simulink model "eCS_Old_Algo_And_Tests"  (R2015b)
settings: Solver=VariableStepAuto  StartTime=0.0  StopTime=10.0  RelTol=1e-3
values from neighbouring files (symbols this model uses):
  pulsetype = 2    [Parameter_eCS_Algo.m]    (also in run_simulation.m = j; run_simulation_ActiveX.m = j)
  rotation = 0    [Parameter_eCS_Algo.m]
  SubPulseType = 1    [Parameter_eCS_Algo.m]
undefined symbols (not defined in the file or in its folder): ddv, DiscIntNeverNeededParam, ECE_45_ax, ECE_45_ay, ECE_45_time, gmw_roada_x__m_s__, gmw_roada_y__m_s__, gmw_roadtime_2kHz, Heiko_AY, Heiko_AY_time, Meldorf_HindenburgstraAcceleration_x__m_s_2_, Meldorf_HindenburgstraAcceleration_y__m_s_2_, Meldorf_HindenburgstraTime__s_, pulse_FF27, pulse_MPDB, pulse_ODB40, pulse_ODB64, pulse_USNCAP, pulsetime_FF27, pulsetime_MPDB, pulsetime_ODB40, pulsetime_ODB64, pulsetime_USNCAP, VW_416_2kHza_x_2kHz, VW_416_2kHza_y_2kHz, VW_416_2kHztime_2kHz
libraries: tllib x9, simulink x9
(part 8 of 8)

== system eCS_Old_Algo_And_Tests/eCS_Algo_in_g1/Crash Acceleration/Acceleration Clipping/If Action Subsystem ==
  u8Sample : Inport
  u8OldTrigger : Inport  Port=2
  u8OldTrimer : Inport  Port=3
  Action Port : ActionPort
  "Clear Trigger " : Subsystem  TreatAsAtomicUnit=on
  Decrease Timer : Subsystem  TreatAsAtomicUnit=on
  If1 : If  IfExpression=u1
  Logical Operator : Logic  AllPortsSameDT=off  OutDataTypeStr=boolean  mask(TL_LogicalOperator){data={'date',737938.66931099538}}
      settings: DeleteFcn=if exist('delete_tlblock','file')==2,delete_tlblock(gcbh);end  NameChangeFcn=if exist('rename_tlblock','file')==2,rename_tlblock(gcbh);end  OpenFcn=if exist('tl_open_blockdlg','file')==2,tl_open_blockdlg(gcbh);else,open_system(gcbh,'parameter');end
      mask Help: eval(['if exist(''tl_online_help'',''file'') == 2, tl_online_help(''Topic'',''TL_LogicalOperator''),else, web([''jar:file:///'',matlabroot,''/help/toolbox/simulink/help.jar!/slref/' lower(get_param(gcbh,'Blocktype')) '.html''], ''-helpbrowser''),end'])
      mask Display: plot([-0.1, 1.05, NaN, -0.1, 1.05],[.01, .01, NaN, .99, .99]);
  Logical Operator1 : Logic  AllPortsSameDT=off  OutDataTypeStr=boolean  mask(TL_LogicalOperator){data={'date',737938.66931099538}}
      settings: DeleteFcn=if exist('delete_tlblock','file')==2,delete_tlblock(gcbh);end  NameChangeFcn=if exist('rename_tlblock','file')==2,rename_tlblock(gcbh);end  OpenFcn=if exist('tl_open_blockdlg','file')==2,tl_open_blockdlg(gcbh);else,open_system(gcbh,'parameter');end
      mask Help: eval(['if exist(''tl_online_help'',''file'') == 2, tl_online_help(''Topic'',''TL_LogicalOperator''),else, web([''jar:file:///'',matlabroot,''/help/toolbox/simulink/help.jar!/slref/' lower(get_param(gcbh,'Blocktype')) '.html''], ''-helpbrowser''),end'])
      mask Display: plot([-0.1, 1.05, NaN, -0.1, 1.05],[.01, .01, NaN, .99, .99]);
  MaxSample2 : Constant  Value=ddv('eCS_CFG/CRASH_SAMPLES_NB')  mask(TL_Constant){data={'output',{'variable','eCS_CFG/CRASH_SAMPLES_NB'},'date',737951.42481170141}}
      settings: CopyFcn=if exist('tl_reset_reviewflag') == 2, tl_reset_reviewflag(gcbh); end  DeleteFcn=if exist('delete_tlblock','file')==2,delete_tlblock(gcbh);end  NameChangeFcn=if exist('rename_tlblock','file')==2,rename_tlblock(gcbh);end  OpenFcn=if exist('tl_open_blockdlg','file')==2,tl_open_blockdlg(gcbh);else,open_system(gcbh,'parameter');end
      mask Help: eval(['if exist(''tl_online_help'',''file'') == 2, tl_online_help(''Topic'',''TL_Constant''),else, web([''jar:file:///'',matlabroot,''/help/toolbox/simulink/help.jar!/slref/' lower(get_param(gcbh,'Blocktype')) '.html''], ''-helpbrowser''),end'])
      mask Display: plot([-0.1, 1.05, NaN, -0.1, 1.05],[.01, .01, NaN, .99, .99]);
  MaxSample3 : Constant  mask(TL_Constant){data={'date',737938.66834370373}}
      settings: CopyFcn=if exist('tl_reset_reviewflag') == 2, tl_reset_reviewflag(gcbh); end  DeleteFcn=if exist('delete_tlblock','file')==2,delete_tlblock(gcbh);end  NameChangeFcn=if exist('rename_tlblock','file')==2,rename_tlblock(gcbh);end  OpenFcn=if exist('tl_open_blockdlg','file')==2,tl_open_blockdlg(gcbh);else,open_system(gcbh,'parameter');end
      mask Help: eval(['if exist(''tl_online_help'',''file'') == 2, tl_online_help(''Topic'',''TL_Constant''),else, web([''jar:file:///'',matlabroot,''/help/toolbox/simulink/help.jar!/slref/' lower(get_param(gcbh,'Blocktype')) '.html''], ''-helpbrowser''),end'])
      mask Display: plot([-0.1, 1.05, NaN, -0.1, 1.05],[.01, .01, NaN, .99, .99]);
  MaxSample4 : Constant  Value=0  mask(TL_Constant){data={'date',737938.62249356485}}
      settings: CopyFcn=if exist('tl_reset_reviewflag') == 2, tl_reset_reviewflag(gcbh); end  DeleteFcn=if exist('delete_tlblock','file')==2,delete_tlblock(gcbh);end  NameChangeFcn=if exist('rename_tlblock','file')==2,rename_tlblock(gcbh);end  OpenFcn=if exist('tl_open_blockdlg','file')==2,tl_open_blockdlg(gcbh);else,open_system(gcbh,'parameter');end
      mask Help: eval(['if exist(''tl_online_help'',''file'') == 2, tl_online_help(''Topic'',''TL_Constant''),else, web([''jar:file:///'',matlabroot,''/help/toolbox/simulink/help.jar!/slref/' lower(get_param(gcbh,'Blocktype')) '.html''], ''-helpbrowser''),end'])
      mask Display: plot([-0.1, 1.05, NaN, -0.1, 1.05],[.01, .01, NaN, .99, .99]);
  Merge : Merge  InitialOutput=0  mask(TL_Merge){data={'date',737951.61381224543}}
      settings: CopyFcn=if exist('tl_reset_reviewflag') == 2, tl_reset_reviewflag(gcbh); end  DeleteFcn=if exist('delete_tlblock','file')==2,delete_tlblock(gcbh);end  NameChangeFcn=if exist('rename_tlblock','file')==2,rename_tlblock(gcbh);end  OpenFcn=if exist('tl_open_blockdlg','file')==2,tl_open_blockdlg(gcbh);else,open_system(gcbh,'parameter');end
      mask Help: eval(['if exist(''tl_online_help'',''file'') == 2, tl_online_help(''Topic'',''TL_Merge''),else, web([''jar:file:///'',matlabroot,''/help/toolbox/simulink/help.jar!/slref/' lower(get_param(gcbh,'Blocktype')) '.html''], ''-helpbrowser''),end'])
      mask Display: plot([-0.1, 1.05, NaN, -0.1, 1.05],[.01, .01, NaN, .99, .99]);
  Merge1 : Merge  InitialOutput=0  mask(TL_Merge){data={'date',737951.6139147107}}
      settings: CopyFcn=if exist('tl_reset_reviewflag') == 2, tl_reset_reviewflag(gcbh); end  DeleteFcn=if exist('delete_tlblock','file')==2,delete_tlblock(gcbh);end  NameChangeFcn=if exist('rename_tlblock','file')==2,rename_tlblock(gcbh);end  OpenFcn=if exist('tl_open_blockdlg','file')==2,tl_open_blockdlg(gcbh);else,open_system(gcbh,'parameter');end
      mask Help: eval(['if exist(''tl_online_help'',''file'') == 2, tl_online_help(''Topic'',''TL_Merge''),else, web([''jar:file:///'',matlabroot,''/help/toolbox/simulink/help.jar!/slref/' lower(get_param(gcbh,'Blocktype')) '.html''], ''-helpbrowser''),end'])
      mask Display: plot([-0.1, 1.05, NaN, -0.1, 1.05],[.01, .01, NaN, .99, .99]);
  Relational Operator2 : RelationalOperator  Operator=<  OutDataTypeStr=boolean  mask(TL_RelationalOperator){data={'date',737938.66802540515}}
      settings: DeleteFcn=if exist('delete_tlblock','file')==2,delete_tlblock(gcbh);end  NameChangeFcn=if exist('rename_tlblock','file')==2,rename_tlblock(gcbh);end  OpenFcn=if exist('tl_open_blockdlg','file')==2,tl_open_blockdlg(gcbh);else,open_system(gcbh,'parameter');end
      mask Help: eval(['if exist(''tl_online_help'',''file'') == 2, tl_online_help(''Topic'',''TL_RelationalOperator''),else, web([''jar:file:///'',matlabroot,''/help/toolbox/simulink/help.jar!/slref/' lower(get_param(gcbh,'Blocktype')) '.html''], ''-helpbrowser''),end'])
      mask Display: plot([-0.1, 1.05, NaN, -0.1, 1.05],[.01, .01, NaN, .99, .99]);
  Relational Operator3 : RelationalOperator  Operator===  OutDataTypeStr=boolean  mask(TL_RelationalOperator){data={'date',737938.62190350692}}
      settings: DeleteFcn=if exist('delete_tlblock','file')==2,delete_tlblock(gcbh);end  NameChangeFcn=if exist('rename_tlblock','file')==2,rename_tlblock(gcbh);end  OpenFcn=if exist('tl_open_blockdlg','file')==2,tl_open_blockdlg(gcbh);else,open_system(gcbh,'parameter');end
      mask Help: eval(['if exist(''tl_online_help'',''file'') == 2, tl_online_help(''Topic'',''TL_RelationalOperator''),else, web([''jar:file:///'',matlabroot,''/help/toolbox/simulink/help.jar!/slref/' lower(get_param(gcbh,'Blocktype')) '.html''], ''-helpbrowser''),end'])
      mask Display: plot([-0.1, 1.05, NaN, -0.1, 1.05],[.01, .01, NaN, .99, .99]);
  Relational Operator4 : RelationalOperator  Operator===  OutDataTypeStr=boolean  mask(TL_RelationalOperator){data={'date',737938.66923611111}}
      settings: DeleteFcn=if exist('delete_tlblock','file')==2,delete_tlblock(gcbh);end  NameChangeFcn=if exist('rename_tlblock','file')==2,rename_tlblock(gcbh);end  OpenFcn=if exist('tl_open_blockdlg','file')==2,tl_open_blockdlg(gcbh);else,open_system(gcbh,'parameter');end
      mask Help: eval(['if exist(''tl_online_help'',''file'') == 2, tl_online_help(''Topic'',''TL_RelationalOperator''),else, web([''jar:file:///'',matlabroot,''/help/toolbox/simulink/help.jar!/slref/' lower(get_param(gcbh,'Blocktype')) '.html''], ''-helpbrowser''),end'])
      mask Display: plot([-0.1, 1.05, NaN, -0.1, 1.05],[.01, .01, NaN, .99, .99]);
  u8Trigger : Outport  InitialOutput=0
  u8Timer : Outport  Port=2  InitialOutput=0
  wires:
  If1/1 -> "Clear Trigger "/Action
  u8Sample/1 -> Relational Operator2/1
  MaxSample2/1 -> Relational Operator2/2
  u8OldTrigger/1 -> Decrease Timer/2(u8OldTrigger), Relational Operator3/2
  MaxSample3/1 -> Relational Operator3/1
  MaxSample4/1 -> Relational Operator4/2
  Relational Operator2/1 -> Logical Operator/1
  Relational Operator3/1 -> Logical Operator/2
  Relational Operator4/1 -> Logical Operator1/2
  Logical Operator/1 -> Logical Operator1/1
  Logical Operator1/1 -> If1/1
  If1/2 -> Decrease Timer/Action
  u8OldTrimer/1 -> "Clear Trigger "/1(u8OldTimer), Relational Operator4/1, Decrease Timer/1(u8OldTimer)
  Merge/1 -> u8Trigger/1
  "Clear Trigger "/1(Trigger) -> Merge/1
  Merge1/1 -> u8Timer/1
  Decrease Timer/1(u8Timer) -> Merge1/1
  Decrease Timer/2(Trigger) -> Merge/2
  "Clear Trigger "/2(u8Timer) -> Merge1/2

== system eCS_Old_Algo_And_Tests/eCS_Algo_in_g1/Crash Acceleration/Acceleration Clipping/Reset timer ==
  Action Port : ActionPort
  HoldingTime : Constant  Value=ddv('eCS_CFG/CRASH_HOLDING_TMR')  mask(TL_Constant){data={'output',{'variable','eCS_CFG/CRASH_HOLDING_TMR'},'date',737951.42743017361}}
      settings: CopyFcn=if exist('tl_reset_reviewflag') == 2, tl_reset_reviewflag(gcbh); end  DeleteFcn=if exist('delete_tlblock','file')==2,delete_tlblock(gcbh);end  NameChangeFcn=if exist('rename_tlblock','file')==2,rename_tlblock(gcbh);end  OpenFcn=if exist('tl_open_blockdlg','file')==2,tl_open_blockdlg(gcbh);else,open_system(gcbh,'parameter');end
      mask Help: eval(['if exist(''tl_online_help'',''file'') == 2, tl_online_help(''Topic'',''TL_Constant''),else, web([''jar:file:///'',matlabroot,''/help/toolbox/simulink/help.jar!/slref/' lower(get_param(gcbh,'Blocktype')) '.html''], ''-helpbrowser''),end'])
      mask Display: plot([-0.1, 1.05, NaN, -0.1, 1.05],[.01, .01, NaN, .99, .99]);
  HoldingTime1 : Constant  mask(TL_Constant){data={'date',737938.66696515051}}
      settings: CopyFcn=if exist('tl_reset_reviewflag') == 2, tl_reset_reviewflag(gcbh); end  DeleteFcn=if exist('delete_tlblock','file')==2,delete_tlblock(gcbh);end  NameChangeFcn=if exist('rename_tlblock','file')==2,rename_tlblock(gcbh);end  OpenFcn=if exist('tl_open_blockdlg','file')==2,tl_open_blockdlg(gcbh);else,open_system(gcbh,'parameter');end
      mask Help: eval(['if exist(''tl_online_help'',''file'') == 2, tl_online_help(''Topic'',''TL_Constant''),else, web([''jar:file:///'',matlabroot,''/help/toolbox/simulink/help.jar!/slref/' lower(get_param(gcbh,'Blocktype')) '.html''], ''-helpbrowser''),end'])
      mask Display: plot([-0.1, 1.05, NaN, -0.1, 1.05],[.01, .01, NaN, .99, .99]);
  u8Timer : Outport  InitialOutput=0
  u8Trigger : Outport  Port=2  InitialOutput=1
  wires:
  HoldingTime/1 -> u8Timer/1
  HoldingTime1/1 -> u8Trigger/1

== system eCS_Old_Algo_And_Tests/eCS_Algo_in_g/Crash Acceleration/Acceleration Clipping/If Action Subsystem/Clear Trigger  ==
  u8OldTimer : Inport
  Action Port : ActionPort
  Constant1 : Constant  Value=0  mask(TL_Constant){data={'date',737938.68007521995}}
      settings: CopyFcn=if exist('tl_reset_reviewflag') == 2, tl_reset_reviewflag(gcbh); end  DeleteFcn=if exist('delete_tlblock','file')==2,delete_tlblock(gcbh);end  NameChangeFcn=if exist('rename_tlblock','file')==2,rename_tlblock(gcbh);end  OpenFcn=if exist('tl_open_blockdlg','file')==2,tl_open_blockdlg(gcbh);else,open_system(gcbh,'parameter');end
      mask Help: eval(['if exist(''tl_online_help'',''file'') == 2, tl_online_help(''Topic'',''TL_Constant''),else, web([''jar:file:///'',matlabroot,''/help/toolbox/simulink/help.jar!/slref/' lower(get_param(gcbh,'Blocktype')) '.html''], ''-helpbrowser''),end'])
      mask Display: plot([-0.1, 1.05, NaN, -0.1, 1.05],[.01, .01, NaN, .99, .99]);
  Trigger : Outport  InitialOutput=0
  u8Timer : Outport  Port=2  InitialOutput=0
  wires:
  Constant1/1 -> Trigger/1
  u8OldTimer/1 -> u8Timer/1

== system eCS_Old_Algo_And_Tests/eCS_Algo_in_g/Crash Acceleration/Acceleration Clipping/If Action Subsystem/Decrease Timer ==
  u8OldTimer : Inport
  u8OldTrigger : Inport  Port=2
  Action Port : ActionPort
  Constant : Constant  mask(TL_Constant){data={'date',737938.67253848375}}
      settings: CopyFcn=if exist('tl_reset_reviewflag') == 2, tl_reset_reviewflag(gcbh); end  DeleteFcn=if exist('delete_tlblock','file')==2,delete_tlblock(gcbh);end  NameChangeFcn=if exist('rename_tlblock','file')==2,rename_tlblock(gcbh);end  OpenFcn=if exist('tl_open_blockdlg','file')==2,tl_open_blockdlg(gcbh);else,open_system(gcbh,'parameter');end
      mask Help: eval(['if exist(''tl_online_help'',''file'') == 2, tl_online_help(''Topic'',''TL_Constant''),else, web([''jar:file:///'',matlabroot,''/help/toolbox/simulink/help.jar!/slref/' lower(get_param(gcbh,'Blocktype')) '.html''], ''-helpbrowser''),end'])
      mask Display: plot([-0.1, 1.05, NaN, -0.1, 1.05],[.01, .01, NaN, .99, .99]);
  Constant1 : Constant  Value=0  mask(TL_Constant){data={'date',737938.6727367593}}
      settings: CopyFcn=if exist('tl_reset_reviewflag') == 2, tl_reset_reviewflag(gcbh); end  DeleteFcn=if exist('delete_tlblock','file')==2,delete_tlblock(gcbh);end  NameChangeFcn=if exist('rename_tlblock','file')==2,rename_tlblock(gcbh);end  OpenFcn=if exist('tl_open_blockdlg','file')==2,tl_open_blockdlg(gcbh);else,open_system(gcbh,'parameter');end
      mask Help: eval(['if exist(''tl_online_help'',''file'') == 2, tl_online_help(''Topic'',''TL_Constant''),else, web([''jar:file:///'',matlabroot,''/help/toolbox/simulink/help.jar!/slref/' lower(get_param(gcbh,'Blocktype')) '.html''], ''-helpbrowser''),end'])
      mask Display: plot([-0.1, 1.05, NaN, -0.1, 1.05],[.01, .01, NaN, .99, .99]);
  HoldingTimer : Switch  Criteria=u2 ~= 0  mask(TL_Switch){data={'output',{'type','UInt16'},'date',737996.37411469908}}
      settings: CopyFcn=if exist('tl_reset_reviewflag') == 2, tl_reset_reviewflag(gcbh); end  DeleteFcn=if exist('delete_tlblock','file')==2,delete_tlblock(gcbh);end  NameChangeFcn=if exist('rename_tlblock','file')==2,rename_tlblock(gcbh);end  OpenFcn=if exist('tl_open_blockdlg','file')==2,tl_open_blockdlg(gcbh);else,open_system(gcbh,'parameter');end
      mask Help: eval(['if exist(''tl_online_help'',''file'') == 2, tl_online_help(''Topic'',''TL_Switch''),else, web([''jar:file:///'',matlabroot,''/help/toolbox/simulink/help.jar!/slref/' lower(get_param(gcbh,'Blocktype')) '.html''], ''-helpbrowser''),end'])
      mask Display: plot([-0.1, 1.05, NaN, -0.1, 1.05],[.01, .01, NaN, .99, .99]);
  Sum : Sum  Inputs=+-  mask(TL_Sum){data={'output',{'type','UInt16'},'date',737996.37424137734}}
      settings: CopyFcn=if exist('tl_reset_reviewflag') == 2, tl_reset_reviewflag(gcbh); end  DeleteFcn=if exist('delete_tlblock','file')==2,delete_tlblock(gcbh);end  NameChangeFcn=if exist('rename_tlblock','file')==2,rename_tlblock(gcbh);end  OpenFcn=if exist('tl_open_blockdlg','file')==2,tl_open_blockdlg(gcbh);else,open_system(gcbh,'parameter');end
      mask Help: eval(['if exist(''tl_online_help'',''file'') == 2, tl_online_help(''Topic'',''TL_Sum''),else, web([''jar:file:///'',matlabroot,''/help/toolbox/simulink/help.jar!/slref/' lower(get_param(gcbh,'Blocktype')) '.html''], ''-helpbrowser''),end'])
      mask Display: plot([-0.1, 1.05, NaN, -0.1, 1.05],[.01, .01, NaN, .99, .99]);
  u8Timer : Outport  InitialOutput=0
  Trigger : Outport  Port=2  InitialOutput=0
  wires:
  u8OldTimer/1 -> Sum/1, HoldingTimer/2
  HoldingTimer/1 -> u8Timer/1
  Constant/1 -> Sum/2
  Sum/1 -> HoldingTimer/1
  Constant1/1 -> HoldingTimer/3
  u8OldTrigger/1 -> Trigger/1

== system eCS_Old_Algo_And_Tests/eCS_Algo_in_g1/Crash Acceleration/Acceleration Clipping/If Action Subsystem/Clear Trigger  ==
  u8OldTimer : Inport
  Action Port : ActionPort
  Constant1 : Constant  Value=0  mask(TL_Constant){data={'date',737938.68007521995}}
      settings: CopyFcn=if exist('tl_reset_reviewflag') == 2, tl_reset_reviewflag(gcbh); end  DeleteFcn=if exist('delete_tlblock','file')==2,delete_tlblock(gcbh);end  NameChangeFcn=if exist('rename_tlblock','file')==2,rename_tlblock(gcbh);end  OpenFcn=if exist('tl_open_blockdlg','file')==2,tl_open_blockdlg(gcbh);else,open_system(gcbh,'parameter');end
      mask Help: eval(['if exist(''tl_online_help'',''file'') == 2, tl_online_help(''Topic'',''TL_Constant''),else, web([''jar:file:///'',matlabroot,''/help/toolbox/simulink/help.jar!/slref/' lower(get_param(gcbh,'Blocktype')) '.html''], ''-helpbrowser''),end'])
      mask Display: plot([-0.1, 1.05, NaN, -0.1, 1.05],[.01, .01, NaN, .99, .99]);
  Trigger : Outport  InitialOutput=0
  u8Timer : Outport  Port=2  InitialOutput=0
  wires:
  Constant1/1 -> Trigger/1
  u8OldTimer/1 -> u8Timer/1

== system eCS_Old_Algo_And_Tests/eCS_Algo_in_g1/Crash Acceleration/Acceleration Clipping/If Action Subsystem/Decrease Timer ==
  u8OldTimer : Inport
  u8OldTrigger : Inport  Port=2
  Action Port : ActionPort
  Constant : Constant  mask(TL_Constant){data={'date',737938.67253848375}}
      settings: CopyFcn=if exist('tl_reset_reviewflag') == 2, tl_reset_reviewflag(gcbh); end  DeleteFcn=if exist('delete_tlblock','file')==2,delete_tlblock(gcbh);end  NameChangeFcn=if exist('rename_tlblock','file')==2,rename_tlblock(gcbh);end  OpenFcn=if exist('tl_open_blockdlg','file')==2,tl_open_blockdlg(gcbh);else,open_system(gcbh,'parameter');end
      mask Help: eval(['if exist(''tl_online_help'',''file'') == 2, tl_online_help(''Topic'',''TL_Constant''),else, web([''jar:file:///'',matlabroot,''/help/toolbox/simulink/help.jar!/slref/' lower(get_param(gcbh,'Blocktype')) '.html''], ''-helpbrowser''),end'])
      mask Display: plot([-0.1, 1.05, NaN, -0.1, 1.05],[.01, .01, NaN, .99, .99]);
  Constant1 : Constant  Value=0  mask(TL_Constant){data={'date',737938.6727367593}}
      settings: CopyFcn=if exist('tl_reset_reviewflag') == 2, tl_reset_reviewflag(gcbh); end  DeleteFcn=if exist('delete_tlblock','file')==2,delete_tlblock(gcbh);end  NameChangeFcn=if exist('rename_tlblock','file')==2,rename_tlblock(gcbh);end  OpenFcn=if exist('tl_open_blockdlg','file')==2,tl_open_blockdlg(gcbh);else,open_system(gcbh,'parameter');end
      mask Help: eval(['if exist(''tl_online_help'',''file'') == 2, tl_online_help(''Topic'',''TL_Constant''),else, web([''jar:file:///'',matlabroot,''/help/toolbox/simulink/help.jar!/slref/' lower(get_param(gcbh,'Blocktype')) '.html''], ''-helpbrowser''),end'])
      mask Display: plot([-0.1, 1.05, NaN, -0.1, 1.05],[.01, .01, NaN, .99, .99]);
  HoldingTimer : Switch  Criteria=u2 ~= 0  mask(TL_Switch){data={'output',{'type','UInt16'},'date',737996.37411469908}}
      settings: CopyFcn=if exist('tl_reset_reviewflag') == 2, tl_reset_reviewflag(gcbh); end  DeleteFcn=if exist('delete_tlblock','file')==2,delete_tlblock(gcbh);end  NameChangeFcn=if exist('rename_tlblock','file')==2,rename_tlblock(gcbh);end  OpenFcn=if exist('tl_open_blockdlg','file')==2,tl_open_blockdlg(gcbh);else,open_system(gcbh,'parameter');end
      mask Help: eval(['if exist(''tl_online_help'',''file'') == 2, tl_online_help(''Topic'',''TL_Switch''),else, web([''jar:file:///'',matlabroot,''/help/toolbox/simulink/help.jar!/slref/' lower(get_param(gcbh,'Blocktype')) '.html''], ''-helpbrowser''),end'])
      mask Display: plot([-0.1, 1.05, NaN, -0.1, 1.05],[.01, .01, NaN, .99, .99]);
  Sum : Sum  Inputs=+-  mask(TL_Sum){data={'output',{'type','UInt16'},'date',737996.37424137734}}
      settings: CopyFcn=if exist('tl_reset_reviewflag') == 2, tl_reset_reviewflag(gcbh); end  DeleteFcn=if exist('delete_tlblock','file')==2,delete_tlblock(gcbh);end  NameChangeFcn=if exist('rename_tlblock','file')==2,rename_tlblock(gcbh);end  OpenFcn=if exist('tl_open_blockdlg','file')==2,tl_open_blockdlg(gcbh);else,open_system(gcbh,'parameter');end
      mask Help: eval(['if exist(''tl_online_help'',''file'') == 2, tl_online_help(''Topic'',''TL_Sum''),else, web([''jar:file:///'',matlabroot,''/help/toolbox/simulink/help.jar!/slref/' lower(get_param(gcbh,'Blocktype')) '.html''], ''-helpbrowser''),end'])
      mask Display: plot([-0.1, 1.05, NaN, -0.1, 1.05],[.01, .01, NaN, .99, .99]);
  u8Timer : Outport  InitialOutput=0
  Trigger : Outport  Port=2  InitialOutput=0
  wires:
  u8OldTimer/1 -> Sum/1, HoldingTimer/2
  HoldingTimer/1 -> u8Timer/1
  Constant/1 -> Sum/2
  Sum/1 -> HoldingTimer/1
  Constant1/1 -> HoldingTimer/3
  u8OldTrigger/1 -> Trigger/1

== matlab function eCS_Old_Algo_And_Tests/eCS Algo new/aceleration clipping trigger ==
  settings: updateMethod=DISCRETE
  data: trigger_out output; pulse_in input; triggertime output; time input; no_of_samples input; a_threshold input
function [trigger_out , triggertime]     = acceleration_clipping_trigger(pulse_in, time, no_of_samples, a_threshold)
%Inputthe pulse signal and count the number of subsequent samples above the
%acceleration threshold - when the numer of allowed samples are reached,
%then the trigger_out goes from 1 to 0 for a certain hold-time
%intention is to detect a crahs-pulse a.s.a.p when the acceleration signal
%excceeds a certain threshold

%local variable declaration
persistent trigger_intern
persistent triggertime_intern
persistent samples_counter


% Initialisation
if isempty(trigger_intern)
   trigger_intern=0;
   triggertime_intern = 0 ;
   samples_counter = 0 ;   
end


%main
if pulse_in>=a_threshold
    samples_counter = samples_counter+1 ;
else
    samples_counter=0;
end



if  and( samples_counter>=no_of_samples , trigger_intern==0)
    trigger_intern=1;
    triggertime_intern=time*1000;
end

if and ( and( samples_counter<no_of_samples , trigger_intern==1) , (time-(triggertime_intern/1000)) > 0.1 )
    trigger_intern=0;
end
% Output
trigger_out=trigger_intern;
triggertime=triggertime_intern;

== matlab function eCS_Old_Algo_And_Tests/eCS Algo new/Trigger_hold_time ==
  data: trigger_in input; trigger_out output; time input; time_delay input
function trigger_out    = Trigger_hold_time(trigger_in,time,time_delay)
%no impact on trigger change from 0 to 1 (-->locking)
%delays the time for the trigger signal from 1 to 0 (-->unlocking) to avoid
%too many subsequent locking in a certain time

%local variable declaration
persistent time_store
persistent trigger_intern

% Initialisation
if isempty(time_store)
   time_store = 0 ;
   trigger_intern = 0 ;   
end

% main
if trigger_in==1 ;
    time_store=time;
    trigger_intern=trigger_in;
end
if time>=(time_store+ (time_delay/1000) );
    trigger_intern=trigger_in;
end

% Output
trigger_out=trigger_intern;

== matlab function eCS_Old_Algo_And_Tests/eCS Algo new1/Trigger_hold_time ==
  data: trigger_in input; trigger_out output; time input; time_delay input
function trigger_out    = Trigger_hold_time(trigger_in,time,time_delay)
%no impact on trigger change from 0 to 1 (-->locking)
%delays the time for the trigger signal from 1 to 0 (-->unlocking) to avoid
%too many subsequent locking in a certain time

%local variable declaration
persistent time_store
persistent trigger_intern

% Initialisation
if isempty(time_store)
   time_store = 0 ;
   trigger_intern = 0 ;   
end

% main
if trigger_in==1 ;
    time_store=time;
    trigger_intern=trigger_in;
end
if time>=(time_store+ (time_delay/1000) );
    trigger_intern=trigger_in;
end

% Output
trigger_out=trigger_intern;

== matlab function eCS_Old_Algo_And_Tests/eCS Algo new1/aceleration clipping trigger ==
  settings: updateMethod=DISCRETE
  data: trigger_out output; pulse_in input; triggertime output; time input; no_of_samples input; a_threshold input
function [trigger_out , triggertime]     = acceleration_clipping_trigger(pulse_in, time, no_of_samples, a_threshold)
%Inputthe pulse signal and count the number of subsequent samples above the
%acceleration threshold - when the numer of allowed samples are reached,
%then the trigger_out goes from 1 to 0 for a certain hold-time
%intention is to detect a crahs-pulse a.s.a.p when the acceleration signal
%excceeds a certain threshold

%local variable declaration
persistent trigger_intern
persistent triggertime_intern
persistent samples_counter


% Initialisation
if isempty(trigger_intern)
   trigger_intern=0;
   triggertime_intern = 0 ;
   samples_counter = 0 ;   
end


%main
if pulse_in>=a_threshold
    samples_counter = samples_counter+1 ;
else
    samples_counter=0;
end



if  and( samples_counter>=no_of_samples , trigger_intern==0)
    trigger_intern=1;
    triggertime_intern=time*1000;
end

if and ( and( samples_counter<no_of_samples , trigger_intern==1) , (time-(triggertime_intern/1000)) > 0.1 )
    trigger_intern=0;
end
% Output
trigger_out=trigger_intern;
triggertime=triggertime_intern;
